simulink model "AlarmConditionEnable"  (R2020b)
settings: Solver=VariableStepAuto  StartTime=0.0  StopTime=100  RelTol=1e-3
undefined symbols (not defined in the file): sigbuilder_block
settings Model: Creator=99003727  LastModifiedBy=99003727

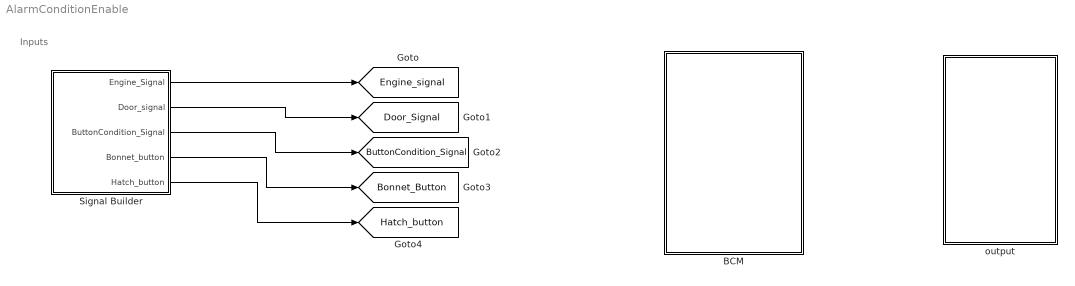
== system AlarmConditionEnable ==
  note: Inputs
  BCM : Subsystem
  Signal Builder : Subsystem  Tag=STV Subsys  LoadFcn=sigbuilder_block('load',[437.6 199.2 550.4 400 ]);  StartFcn=sigbuilder_block('start');  StopFcn=sigbuilder_block('stop');  ClipboardFcn=sigbuilder_block('clipboard');  mask(Sigbuilder block){tuvar=[0:10]}
      mask help: Simulink:masks:SigbuilderBlock_MD
      mask init:
      | if ~strcmp(get_param(bdroot(gcbh),'SimulationStatus'),'stopped') tuvar = sigbuilder_block('maskInit'); end
      settings: CopyFcn=sigbuilder_block('copy');  DeleteFcn=sigbuilder_block('delete');  ModelCloseFcn=sigbuilder_block('modelClose');  PreSaveFcn=sigbuilder_block('preSave');  PauseFcn=sigbuilder_block('pause');  ContinueFcn=sigbuilder_block('continue');  NameChangeFcn=sigbuilder_block('namechange');  OpenFcn=sigbuilder_block('open',[437.6 199.2 550.4 400 ]);  CloseFcn=sigbuilder_block('close');
      mask Display: plot(0, 0, 100, 100,[2, 2, 32, 32, 2], [68, 8, 8, 68, 68],[32, 2], [38, 38], [32, 19, 2],[53, 60, 44], [32, 17, 17, 2],[16, 16, 31, 31]);txt = getActiveGroup(gcbh);text(2, 100, txt,'verticalAlignment', 'top');
  output : Subsystem
  tag scope: Bonnet_Button=global, ButtonCondition_Signal=global, Door_Signal=global, Engine_signal=global, Hatch_button=global
  wires:
  Signal Builder/2(Door_signal) -> [Door_Signal]
  Signal Builder/4(Bonnet_button) -> [Bonnet_Button]
  Signal Builder/5(Hatch_button) -> [Hatch_button]
  Signal Builder/3(ButtonCondition_Signal) -> [ButtonCondition_Signal]
  Signal Builder/1(Engine_Signal) -> [Engine_signal]

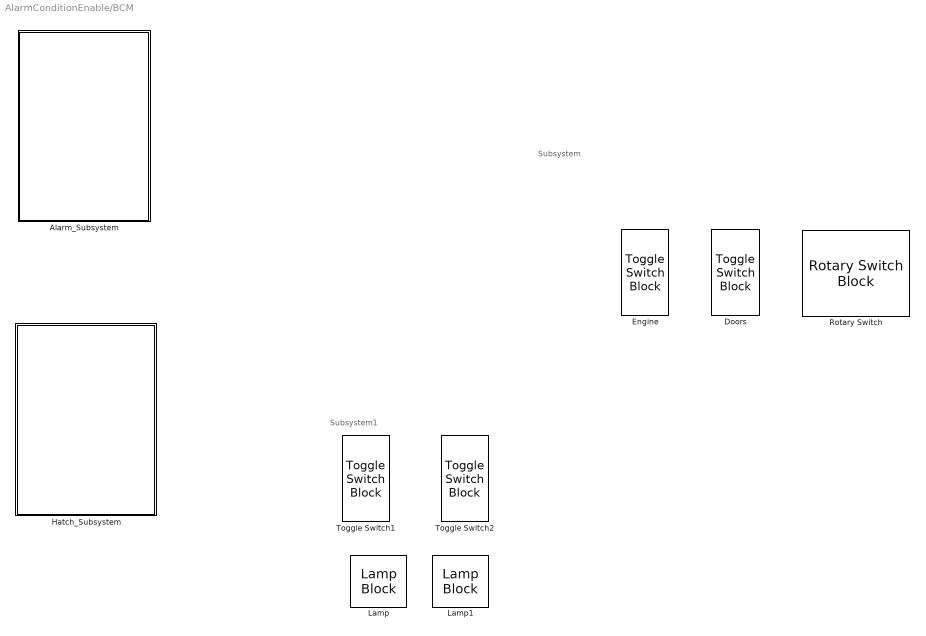
== system AlarmConditionEnable/BCM ==
  note: Subsystem
  note: Subsystem1
  Alarm_Subsystem : Subsystem
  Doors : ToggleSwitchBlock
      settings: Values={{'Off', 'On'}, [0 1]}
  Engine : ToggleSwitchBlock
      settings: Values={{'Off', 'On'}, [0 1]}
  Hatch_Subsystem : Subsystem
  Lamp : LampBlock
  Lamp1 : LampBlock
  Rotary Switch : RotarySwitchBlock
      settings: Values={{'Off', 'Button', 'Double Press'}, [0 1 2]}
  Toggle Switch1 : ToggleSwitchBlock
      settings: Values={{'Bonnet Off', 'Bonnet On'}, [0 1]}
  Toggle Switch2 : ToggleSwitchBlock
      settings: Values={{'Bonnet Off', 'Bonnet On'}, [0 1]}

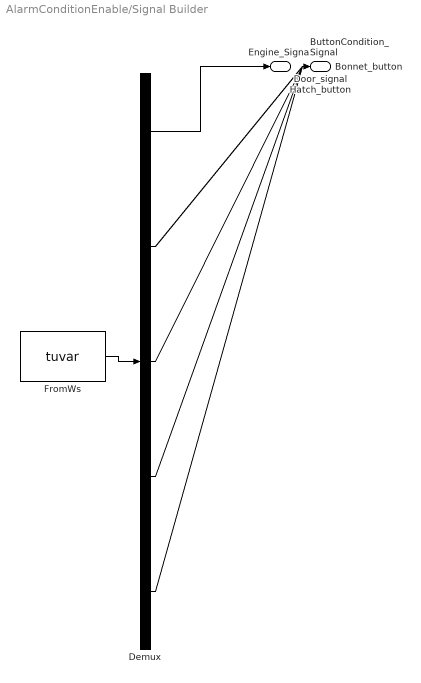
== system AlarmConditionEnable/Signal Builder ==
  Demux : Demux  Tag=STV Demux  Outputs=5
      settings: DisplayOption=none
  FromWs : FromWorkspace  Tag=STV FromWs  VariableName=tuvar
      SigBuilderData=|
      | common.afterFinalStr = 'Extrapolate'
      | common.sampleTime = 0
      | dataSet.timeRange = [0 10]
      | dataSet.name = 'Group 1'
      | sbobj.Groups.Name = 'Group 1'
      | sbobj.Groups.Signals(1).Name = 'Engine_Signal'
      | sbobj.Groups.Signals(1).XData = [0 5 5 10 10 15 15 20 20 25 25 30 30 35 35 40 40 45 45 50 50 55 55 60 60 65 65 70 70 75 75 80 80 85 85 90 90 95 95 100]
      | sbobj.Groups.Signals(1).YData = [0 0 1 1 0 0 1 1 0 0 1 1 0 0 1 1 0 0 1 1 0 0 1 1 0 0 1 1 0 0 1 1 0 0 1 1 0 0 1 1]
      | sbobj.Groups.Signals(2).Name = 'Door_signal'
      | sbobj.Groups.Signals(2).XData = [0 5 5 10 10 15 15 20 20 25 25 30 30 35 35 40 40 45 45 50 50 55 55 60 60 65 65 70 70 75 75 80 80 85 85 90 90 95 95 100]
      | sbobj.Groups.Signals(2).YData = [1 1 0 0 1 1 0 0 1 1 0 0 1 1 0 0 1 1 0 0 1 1 0 0 1 1 0 0 1 1 0 0 1 1 0 0 1 1 0 0]
      | sbobj.Groups.Signals(3).Name = 'ButtonCondition_Signal'
      | sbobj.Groups.Signals(3).XData = [0 5 5 10 15 20 20 25 30 35 35 40 40 45 45 50 50 55 60 60 65 65 70 70 75 75 80 85 90 95 95 100]
      | sbobj.Groups.Signals(3).YData = [0 0 1 2 2 0 1 2 2 0 1 2 0 1 2 0 1 1 1 2 0 1 2 0 1 2 1 1 1 0 1 1]
      | sbobj.Groups.Signals(4).Name = 'Bonnet_button'
      | sbobj.Groups.Signals(4).XData = [0 5 5 10 10 15 15 20 20 25 25 30 30 35 35 40 40 45 45 50 50 55 55 60 60 65 65 70 70 75 75 80 80 85 85 90 90 95 95 100]
      | sbobj.Groups.Signals(4).YData = [0 0 1 1 0 0 1 1 0 0 1 1 0 0 1 1 0 0 1 1 0 0 1 1 0 0 1 1 0 0 1 1 0 0 1 1 0 0 1 1]
      | sbobj.Groups.Signals(5).Name = 'Hatch_button'
      | sbobj.Groups.Signals(5).XData = [0 5 5 10 10 15 15 20 20 25 25 30 30 35 35 40 40 45 45 50 50 55 55 60 60 65 65 70 70 75 75 80 80 85 85 90 90 95 95 100]
      | sbobj.Groups.Signals(5).YData = [1 1 0 0 1 1 0 0 1 1 0 0 1 1 0 0 1 1 0 0 1 1 0 0 1 1 0 0 1 1 0 0 1 1 0 0 1 1 0 0]
  Engine_Signal : Outport  Tag=STV Outport
  Door_signal : Outport  Tag=STV Outport  Port=2
  ButtonCondition_Signal : Outport  Tag=STV Outport  Port=3
  Bonnet_button : Outport  Tag=STV Outport  Port=4
  Hatch_button : Outport  Tag=STV Outport  Port=5
  wires:
  FromWs/1 -> Demux/1
  Demux/1 -> Engine_Signal/1
  Demux/2 -> Door_signal/1
  Demux/3 -> ButtonCondition_Signal/1
  Demux/4 -> Bonnet_button/1
  Demux/5 -> Hatch_button/1

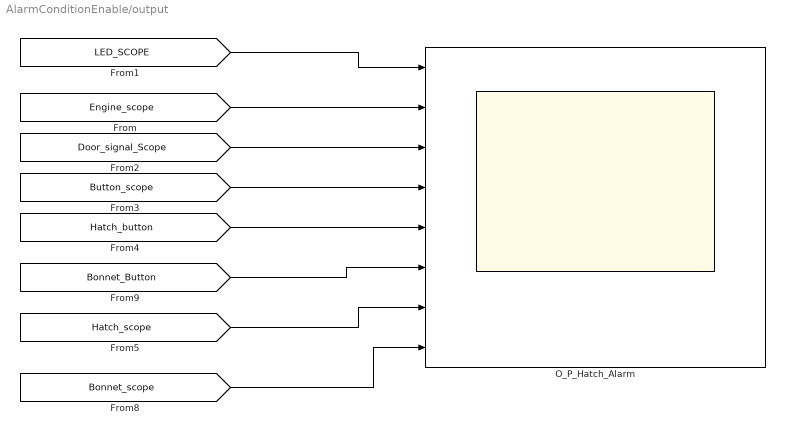
== system AlarmConditionEnable/output ==
  O_P_Hatch_Alarm : Scope  NumInputPorts=8
  wires:
  [LED_SCOPE] -> O_P_Hatch_Alarm/1
  [Engine_scope] -> O_P_Hatch_Alarm/2
  [Door_signal_Scope] -> O_P_Hatch_Alarm/3
  [Button_scope] -> O_P_Hatch_Alarm/4
  [Hatch_button] -> O_P_Hatch_Alarm/5
  [Bonnet_Button] -> O_P_Hatch_Alarm/6
  [Hatch_scope] -> O_P_Hatch_Alarm/7
  [Bonnet_scope] -> O_P_Hatch_Alarm/8

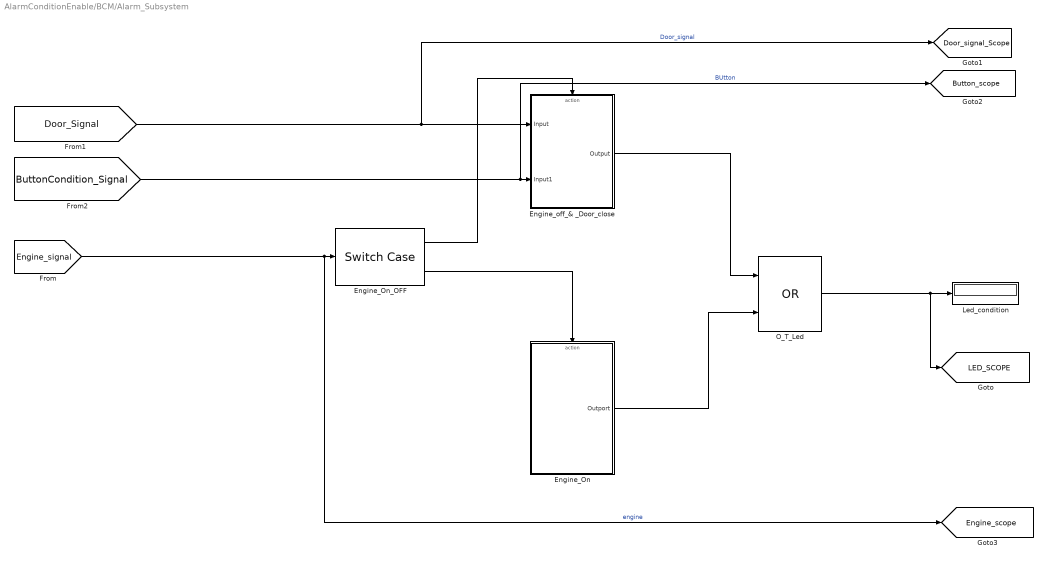
== system AlarmConditionEnable/BCM/Alarm_Subsystem ==
  Engine_On : Subsystem  TreatAsAtomicUnit=on
  Engine_On_OFF : SwitchCase  CaseConditions={0,1}  ShowDefaultCase=off
  Engine_off_& _Door_close : Subsystem  TreatAsAtomicUnit=on
  Led_condition : Display
  O_T_Led : Logic  Operator=OR  IconShape=distinctive  AllPortsSameDT=off  OutDataTypeStr=boolean
  tag scope: Button_scope=global, Door_signal_Scope=global, Engine_scope=global, LED_SCOPE=global
  wires:
  O_T_Led/1 -> [LED_SCOPE], Led_condition/1
  Engine_On_OFF/1 -> Engine_off_& _Door_close/Action
  Engine_On_OFF/2 -> Engine_On/Action
  Engine_On/1(Outport) -> O_T_Led/2
  Engine_off_& _Door_close/1(Output) -> O_T_Led/1
  [Engine_signal] -> [Engine_scope], Engine_On_OFF/1  "engine"
  [Door_Signal] -> [Door_signal_Scope], Engine_off_& _Door_close/1(Input)  "Door_signal"
  [ButtonCondition_Signal] -> [Button_scope], Engine_off_& _Door_close/2(Input1)  "BUtton"

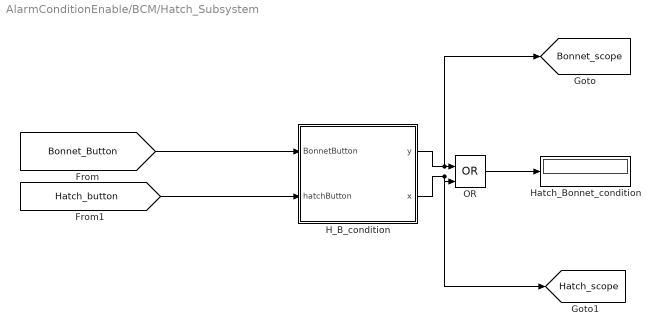
== system AlarmConditionEnable/BCM/Hatch_Subsystem ==
  H_B_condition : Stateflow chart  TreatAsAtomicUnit=on
  Hatch_Bonnet_condition : Display
  OR : Logic  Operator=OR  IconShape=distinctive  AllPortsSameDT=off  OutDataTypeStr=boolean
  tag scope: Bonnet_scope=global, Hatch_scope=global
  wires:
  [Bonnet_Button] -> H_B_condition/1(BonnetButton)
  OR/1 -> Hatch_Bonnet_condition/1
  H_B_condition/1(y) -> [Bonnet_scope], OR/1
  H_B_condition/2(x) -> [Hatch_scope], OR/2
  [Hatch_button] -> H_B_condition/2(hatchButton)

== system AlarmConditionEnable/BCM/Alarm_Subsystem/Engine_On ==
  Action Port : ActionPort  ActionPortLabel=case [ 1 ]:
  Enigine_Off : Constant  Value=0
  Outport : Outport
  wires:
  Enigine_Off/1 -> Outport/1

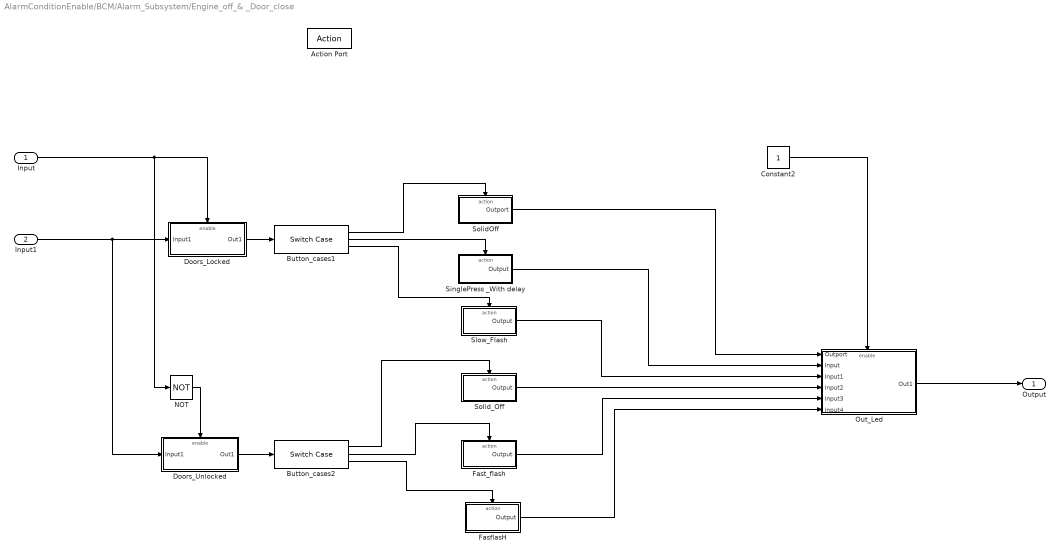
== system AlarmConditionEnable/BCM/Alarm_Subsystem/Engine_off_& _Door_close ==
  Input : Inport
  Input1 : Inport  Port=2
  Action Port : ActionPort  ActionPortLabel=case [ 0 ]:
  " SolidOff" : Subsystem  TreatAsAtomicUnit=on
  Button_cases1 : SwitchCase  CaseConditions={0,1,2}  ShowDefaultCase=off
  Button_cases2 : SwitchCase  CaseConditions={0,1,2}  ShowDefaultCase=off
  Constant2 : Constant
  Doors_Locked : Subsystem  TreatAsAtomicUnit=on
  Doors_Unlocked : Subsystem  TreatAsAtomicUnit=on
  FasflasH : Subsystem  TreatAsAtomicUnit=on
  Fast_flash : Subsystem  TreatAsAtomicUnit=on
  NOT : Logic  Operator=NOT  IconShape=distinctive  AllPortsSameDT=off  OutDataTypeStr=boolean
  Out_Led : Subsystem  TreatAsAtomicUnit=on
  SinglePress _With delay : Subsystem  TreatAsAtomicUnit=on
  Slow_Flash : Subsystem  TreatAsAtomicUnit=on
  Solid_Off : Subsystem  TreatAsAtomicUnit=on
  Output : Outport
  wires:
  Out_Led/1(Out1) -> Output/1
  Button_cases1/1 -> " SolidOff"/Action
  Button_cases1/2 -> SinglePress _With delay/Action
  Button_cases1/3 -> Slow_Flash/Action
  Doors_Locked/1(Out1) -> Button_cases1/1
  NOT/1 -> Doors_Unlocked/Enable
  Doors_Unlocked/1(Out1) -> Button_cases2/1
  Button_cases2/1 -> Solid_Off/Action
  Button_cases2/2 -> Fast_flash/Action
  Button_cases2/3 -> FasflasH/Action
  Constant2/1 -> Out_Led/Enable
  Slow_Flash/1(Output) -> Out_Led/3(Input1)
  Fast_flash/1(Output) -> Out_Led/5(Input3)
  FasflasH/1(Output) -> Out_Led/6(Input4)
  SinglePress _With delay/1(Output) -> Out_Led/2(Input)
  Solid_Off/1(Output) -> Out_Led/4(Input2)
  " SolidOff"/1(Outport) -> Out_Led/1(Outport)
  Input/1 -> NOT/1, Doors_Locked/Enable
  Input1/1 -> Doors_Unlocked/1(Input1), Doors_Locked/1(Input1)

== system AlarmConditionEnable/BCM/Alarm_Subsystem/Engine_off_& _Door_close/ SolidOff ==
  Action Port : ActionPort  ActionPortLabel=case [ 0 ]:
  Constant : Constant  Value=0
  Outport : Outport
  wires:
  Constant/1 -> Outport/1

== system AlarmConditionEnable/BCM/Alarm_Subsystem/Engine_off_& _Door_close/Doors_Locked ==
  Input1 : Inport
  Enable : EnablePort
  Out1 : Outport
  wires:
  Input1/1 -> Out1/1

== system AlarmConditionEnable/BCM/Alarm_Subsystem/Engine_off_& _Door_close/Doors_Unlocked ==
  Input1 : Inport
  Enable : EnablePort
  Out1 : Outport
  wires:
  Input1/1 -> Out1/1

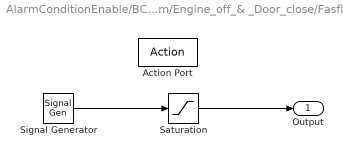
== system AlarmConditionEnable/BCM/Alarm_Subsystem/Engine_off_& _Door_close/FasflasH ==
  Action Port : ActionPort  ActionPortLabel=case [ 2 ]:
  Saturation : Saturate  UpperLimit=1  LowerLimit=0
  Signal Generator : SignalGenerator
  Output : Outport
  wires:
  Saturation/1 -> Output/1
  Signal Generator/1 -> Saturation/1

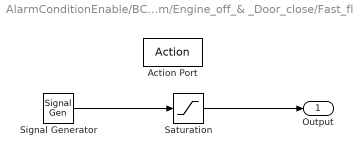
== system AlarmConditionEnable/BCM/Alarm_Subsystem/Engine_off_& _Door_close/Fast_flash ==
  Action Port : ActionPort  ActionPortLabel=case [ 1 ]:
  Saturation : Saturate  UpperLimit=1  LowerLimit=0
  Signal Generator : SignalGenerator  WaveForm=square
  Output : Outport
  wires:
  Saturation/1 -> Output/1
  Signal Generator/1 -> Saturation/1

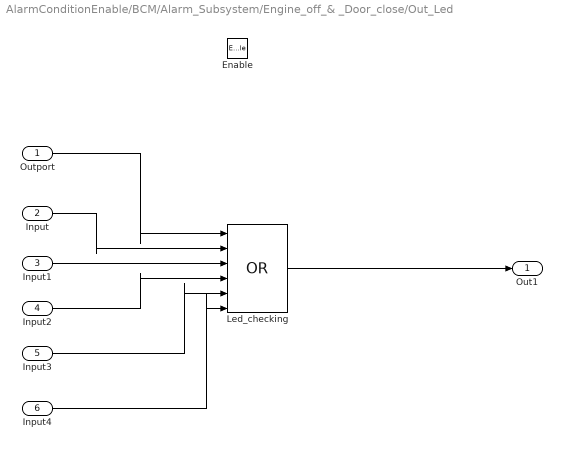
== system AlarmConditionEnable/BCM/Alarm_Subsystem/Engine_off_& _Door_close/Out_Led ==
  Outport : Inport
  Input : Inport  Port=2
  Input1 : Inport  Port=3
  Input2 : Inport  Port=4
  Input3 : Inport  Port=5
  Input4 : Inport  Port=6
  Enable : EnablePort
  Led_checking : Logic  Operator=OR  Inputs=6  IconShape=distinctive  AllPortsSameDT=off  OutDataTypeStr=boolean
  Out1 : Outport
  wires:
  Outport/1 -> Led_checking/1
  Input/1 -> Led_checking/2
  Input1/1 -> Led_checking/3
  Input2/1 -> Led_checking/4
  Input3/1 -> Led_checking/5
  Input4/1 -> Led_checking/6
  Led_checking/1 -> Out1/1

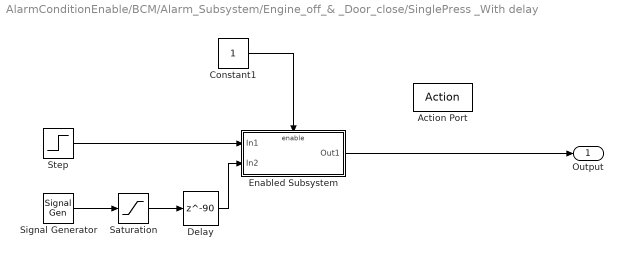
== system AlarmConditionEnable/BCM/Alarm_Subsystem/Engine_off_& _Door_close/SinglePress _With delay ==
  Action Port : ActionPort  ActionPortLabel=case [ 1 ]:
  Constant1 : Constant
  Delay : Delay  DelayLength=90
  Enabled Subsystem : Subsystem  TreatAsAtomicUnit=on
  Saturation : Saturate  UpperLimit=1  LowerLimit=0
  Signal Generator : SignalGenerator  WaveForm=square  Frequency=0.5
  Step : Step  Time=30  Before=1  After=0  SampleTime=0
  Output : Outport
  wires:
  Enabled Subsystem/1(Out1) -> Output/1
  Delay/1 -> Enabled Subsystem/2(In2)
  Saturation/1 -> Delay/1
  Constant1/1 -> Enabled Subsystem/Enable
  Signal Generator/1 -> Saturation/1
  Step/1 -> Enabled Subsystem/1(In1)

== system AlarmConditionEnable/BCM/Alarm_Subsystem/Engine_off_& _Door_close/Slow_Flash ==
  Action Port : ActionPort  ActionPortLabel=case [ 2 ]:
  Saturation : Saturate  UpperLimit=1  LowerLimit=0
  Signal Generator : SignalGenerator  WaveForm=square  Frequency=0.5
  Output : Outport
  wires:
  Saturation/1 -> Output/1
  Signal Generator/1 -> Saturation/1

== system AlarmConditionEnable/BCM/Alarm_Subsystem/Engine_off_& _Door_close/Solid_Off ==
  Action Port : ActionPort  ActionPortLabel=case [ 0 ]:
  Constant : Constant  Value=0
  Output : Outport
  wires:
  Constant/1 -> Output/1

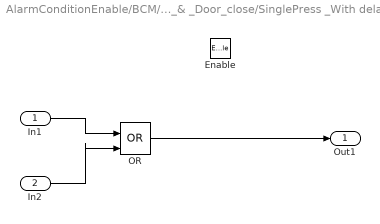
== system AlarmConditionEnable/BCM/Alarm_Subsystem/Engine_off_& _Door_close/SinglePress _With delay/Enabled Subsystem ==
  In1 : Inport
  In2 : Inport  Port=2
  Enable : EnablePort
  OR : Logic  Operator=OR  IconShape=distinctive  AllPortsSameDT=off  OutDataTypeStr=boolean
  Out1 : Outport
  wires:
  In1/1 -> OR/1
  In2/1 -> OR/2
  OR/1 -> Out1/1

== stateflow chart AlarmConditionEnable/BCM/Hatch_Subsystem/H_B_condition ==
  state Hatch
    entry:
    if hatchButton==1
    y=1;
    end
    if BonnetButton==1
    x=1;
    end
  state Hatch_off
    entry:
    if hatchButton==0
    y=0;
    end
    if BonnetButton==0
    x=0;
    end
  (default) -> Hatch
  Hatch -> Hatch_off : [BonnetButton==0||hatchButton==0]
  Hatch_off -> Hatch : [BonnetButton==1||hatchButton==1]
  data: BonnetButton input; hatchButton input; y output; x output
